simulink model "signal_generator"  (R2019b)
settings: Solver=VariableStepAuto  StartTime=0.0  StopTime=10.0  RelTol=1e-3
settings Model: Creator=yango  LastModifiedBy=yango

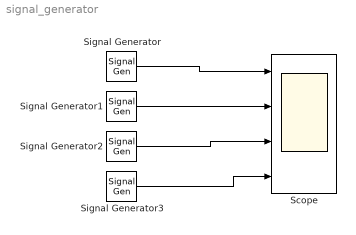
== system signal_generator ==
  Scope : Scope  NumInputPorts=4
  Signal Generator : SignalGenerator  WaveForm=square  Frequency=5  Units=rad/sec
  Signal Generator1 : SignalGenerator  Units=rad/sec
  Signal Generator2 : SignalGenerator  WaveForm=sawtooth  Units=rad/sec
  Signal Generator3 : SignalGenerator  WaveForm=random  Units=rad/sec
  wires:
  Signal Generator/1 -> Scope/1
  Signal Generator1/1 -> Scope/2
  Signal Generator2/1 -> Scope/3
  Signal Generator3/1 -> Scope/4
